simulink model "LoadControl_rev4p2"  (R2024a)
settings: Solver=ode1  StartTime=0.0  StopTime=300  FixedStep=0.001  RelTol=1e-3
undefined symbols (not defined in the file): guxai, K, omega
libraries: SignalEditorBlockLib x2
settings Model: Creator=Hajime.Kondo  LastModifiedBy=Hajime.Kondo

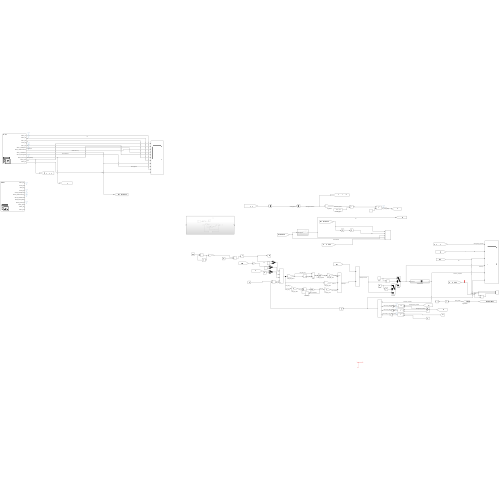
[thumbnail: Simulink's stored preview of the top-level diagram]
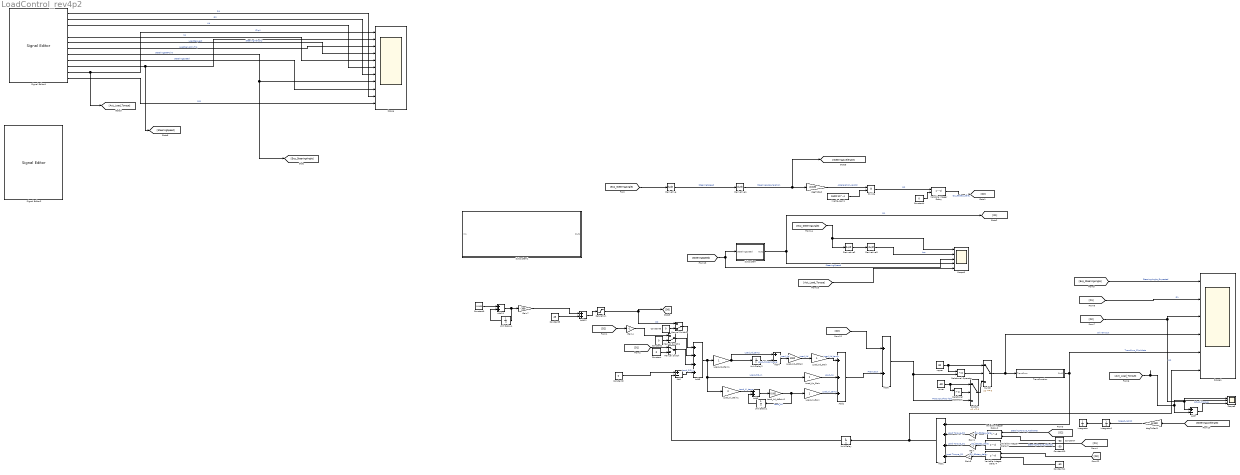
== system LoadControl_rev4p2 ==
  Add : Sum  Inputs=+-
  Add1 : Sum  Inputs=++++
  Add{3,6,11..12} (4 alike) : Sum
  Add2 : Sum  Inputs=+++
  Add4 : Sum  Inputs=+-
  Add5 : Sum  Inputs=++++
  Add7 : Sum  Inputs=+-
  Constant{,1..2,4,6} (5 alike) : Constant  Value=0
  Constant10 : Constant  Value=-50
  Constant11 : Constant  Value=-50
  Constant7 : Constant  Value=-50
  Constant8 : Constant  Value=46
  Constant9 : Constant  Value=0.001
  Derivative{,1..3} (4 alike) : Derivative
  Divide : Product  Inputs=**
  Gain{,1,4..5} (4 alike) : Gain  Gain=-1
  Gain7 : Gain  Gain=-368
  Inertia_kgm1 : Constant  Value=1500*10^-4
  Integrator : Integrator
  Integrator1 : Integrator
  Load_Kd_Gain : Gain
  Load_Kd_Gain1 : Gain
  Load_Kd_dtGain : Gain  Gain=1000
  Load_Kd_dtGain2 : Gain  Gain=0.001
  Load_Ki_Gain : Gain
  Load_Ki_Gain1 : Gain  Gain=0
  Load_Kp_Gain : Gain
  Lower : Constant  Value=-80
  Manual Switch : ManualSwitch
  Manual Switch1 : ManualSwitch  CurrentSetting=0
  Manual Switch2 : ManualSwitch  CurrentSetting=0
  Relational Operator : RelationalOperator  Operator=<=  OutDataTypeStr=boolean  RndMeth=Simplest  InputSameDT=off
  Relational Operator1 : RelationalOperator  OutDataTypeStr=boolean  RndMeth=Simplest  InputSameDT=off
  Saturation : Saturate  UpperLimit=inf  LowerLimit=0
  Scope : Scope  NumInputPorts=11
  Scope1 : Scope  NumInputPorts=6
  Scope3 : Scope  NumInputPorts=5
  Scope6 : Scope  NumInputPorts=3
  Signal Editor1 : SignalEditorBlockLib/Signal Editor  FileName=Simfile.mat  ActiveScenario=SC_rev2  ActiveSignal=data17_D1  IsBus=off  OutputBusObjectStr=Bus: BusObject  SampleTime=0  Interpolate=off  ZeroCross=off  OutputAfterFinalValue=Setting to zero  Unit=inherit  PreserveSignalName=on  ApplySigPropsToAllScenarios=on  ApplySigPropsToAllSignals=off
  Signal Editor2 : SignalEditorBlockLib/Signal Editor  FileName=Simfile.mat  ActiveScenario=SC_rev1  ActiveSignal=data16_Kd  IsBus=off  OutputBusObjectStr=Bus: BusObject  SampleTime=0  Interpolate=off  ZeroCross=off  OutputAfterFinalValue=Setting to zero  Unit=inherit  PreserveSignalName=on  ApplySigPropsToAllScenarios=on  ApplySigPropsToAllSignals=off
  Subsystem : Subsystem
  Subsystem1 : Subsystem
  Switch : Switch  Criteria=u2 ~= 0  SaturateOnIntegerOverflow=off  InputSameDT=off
  Switch1 : Switch  Criteria=u2 ~= 0  SaturateOnIntegerOverflow=off  InputSameDT=off
  TransFunction : Subsystem
  Unit Delay{,1..2,4} (4 alike) : UnitDelay  SampleTime=-1  HasFrameUpgradeWarning=on
  Variable Integer Delay{,2..4} (4 alike) : Delay  DelayLengthSource=Input port
      settings: InputPortMap=u0,p1
  degToRad : Gain  Gain=pi/180
  degToRad1 : Gain  Gain=pi/180
  upper : Constant  Value=80
  wires:
  Signal Editor1/2 -> Scope/7  "D2"
  Signal Editor1/5 -> Scope/5  "Kp"
  Signal Editor1/6 -> Scope/4  "LoadRequest"
  Signal Editor1/7 -> Scope/3  "LoadServoDrvTrq"
  Signal Editor1/10 -> Scope/2, [SteeringSpeed]  "SteeringVelocity"
  Signal Editor1/11 -> [Act_Load_Torque], Scope/1  "ClipX"
  Signal Editor1/8 -> [Exp_SteeringAngle], Scope/8  "SteeringSetPoint"
  Signal Editor1/9 -> Scope/9  "SteeringSpeed"
  ? -> ?
  Variable Integer Delay/1 -> [D2]  "D2_80step_delay"
  [Exp_SteeringAngle] -> Derivative/1
  Add4/1 -> Load_Kd_dtGain/1  "Load_Kd"
  Load_Kp_Gain/1 -> Add2/2  "Load_Kp"
  Lower/1 -> Switch1/1, Relational Operator1/1
  Add3/1 -> Load_Kd_dtGain2/1
  Constant2/1 -> Add/1
  Subsystem/1(Out1) -> Scope3/4, [D1]  "D1"
  Load_Kd_dtGain/1 -> Load_Kd_Gain/1  "Load_Kd"
  Unit Delay/1 -> Add/2
  Relational Operator/1 -> Switch/2
  Manual Switch/1 -> Add5/3
  TransFunction/1(Out1) -> Scope1/5, Add1/1  "TransFunc_ClipXdata"
  Switch1/1 -> Switch/3
  Switch/1 -> Scope1/4, TransFunction/1(TransFunc)  "DriverInput"
  [D2] -> Variable Integer Delay2/1  "SteeringTorque_Acelerate"
  upper/1 -> Switch/1, Relational Operator/1
  Unit Delay2/1 -> Add4/2  "Load_Kd_temp_pre"
  [D2] -> Gain4/1
  [D1] -> Manual Switch/1
  Constant1/1 -> Manual Switch1/2
  [D1] -> Scope1/2  "D1"
  Gain1/1 -> Add1/2  "Load Torque_D2"
  Load_Kd_dtGain2/1 -> Load_Ki_Gain/1, Unit Delay1/1  "Load_Kd"
  Inertia_kgm1/1 -> Divide/2
  Gain/1 -> Add1/3  "Load Torque_D1"
  Add5/1 -> Load_Ki_Gain1/1, Load_Kp_Gain/1, Load_Kd_Gain1/1  "Load_PID_In"
  Integrator1/1 -> Integrator/1
  Unit Delay1/1 -> Add3/2
  [SteeringAcelerate] -> degToRad1/1
  Add7/1 -> Scope6/3
  [Exp_SteeringAngle] -> Scope1/1  "SteeringAngle_Expected"
  Constant8/1 -> Add12/2
  Gain4/1 -> Manual Switch1/1
  Derivative1/1 -> [SteeringAcelerate], degToRad/1  "SteeringAccewleration"
  [D1] -> Variable Integer Delay3/1  "SteeringTorque_Velocity"
  Constant9/1 -> Add11/1
  Gain7/1 -> Add12/1
  degToRad/1 -> Divide/1  "Acceleration_rad/s2"
  Load_Kd_Gain1/1 -> Add4/1, Unit Delay2/1  "Load_Kd_temp"
  Add12/1 -> Saturation/1
  Variable Integer Delay3/1 -> Gain/1  "D2_80step_delay"
  Unit Delay4/1 -> Add11/2
  Load_Ki_Gain/1 -> Add2/3  "Load_Ki_temp"
  degToRad1/1 -> Integrator1/1  "Speed_rad/s2"
  Load_Kd_Gain/1 -> Add2/1  "Load_Kd_temp"
  Constant10/1 -> Variable Integer Delay3/2
  Divide/1 -> Variable Integer Delay/1  "D2"
  Constant7/1 -> Variable Integer Delay2/2
  Variable Integer Delay2/1 -> Gain1/1  "D2_80step_delay"
  Variable Integer Delay4/1 -> Gain5/1  "D2_80step_delay"
  Gain5/1 -> Add1/4  "Load Torque_D1"
  [D0] -> Variable Integer Delay4/1
  Manual Switch1/1 -> Add5/2
  Constant6/1 -> Manual Switch2/2
  Constant11/1 -> Variable Integer Delay4/2
  Add/1 -> Add5/4  "Load_PID_In"
  [Act_Load_Torque] -> Add7/2, Scope6/2  "Actual_Torque"
  Manual Switch2/1 -> Add5/1
  Load_Ki_Gain1/1 -> Add3/1  "Load_Ki_temp"
  Add1/1 -> Scope1/6, Unit Delay/1
  Add11/1 -> Unit Delay4/1, Gain7/1
  Constant/1 -> Manual Switch/2
  [D2] -> Add7/1, Scope6/1, Scope1/3  "D2"
  Relational Operator1/1 -> Switch1/2
  Constant4/1 -> Variable Integer Delay/2
  Saturation/1 -> Manual Switch2/1, [D0]  "D0"
  Add2/1 -> Add6/2  "PIDoutput"
  Add6/1 -> Switch1/3, Relational Operator/2  "PIDoutput+D1+D2"
  [D2] -> Add6/1
  Derivative/1 -> Derivative1/1  "SteeringSpeed"
  [SteeringSpeed] -> Scope3/3, Subsystem/1(SteeringSpeed)  "SteeringSpeed"
  [Act_Load_Torque] -> Scope3/5
  Derivative2/1 -> Derivative3/1
  [Exp_SteeringAngle] -> Derivative2/1, Scope3/1
  Derivative3/1 -> Scope3/2  "Acc"
  Signal Editor1/1 -> Scope/10  "D1"
  Signal Editor1/12 -> Scope/11  "PID"
  Signal Editor1/3 -> Scope/6  "Kd"

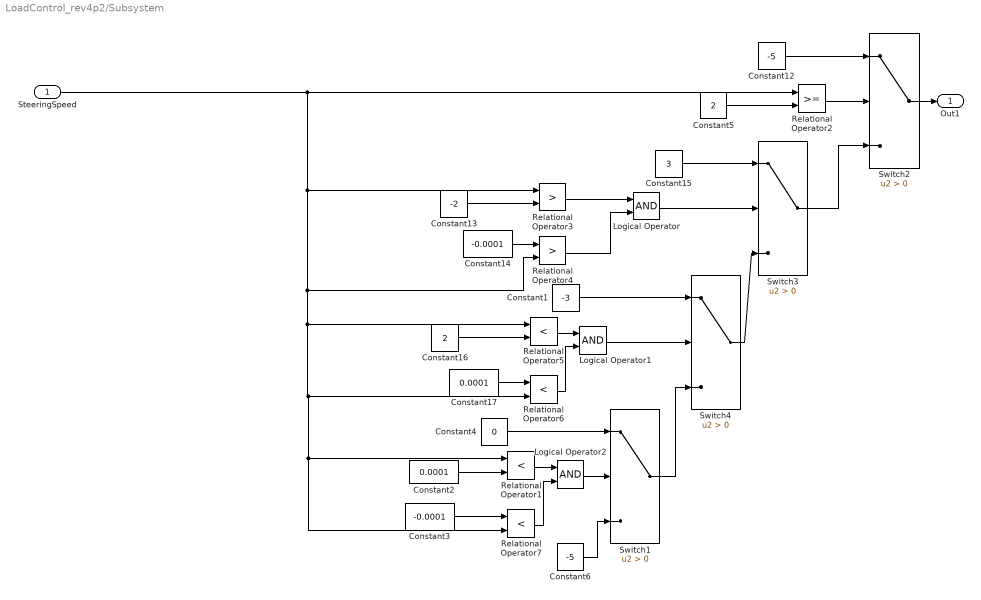
== system LoadControl_rev4p2/Subsystem ==
  SteeringSpeed : Inport
  Constant1 : Constant  Value=-3
  Constant12 : Constant  Value=-5
  Constant13 : Constant  Value=-2
  Constant14 : Constant  Value=-0.0001
  Constant15 : Constant  Value=3
  Constant16 : Constant  Value=2
  Constant17 : Constant  Value=0.0001
  Constant2 : Constant  Value=0.0001
  Constant3 : Constant  Value=-0.0001
  Constant4 : Constant  Value=0
  Constant5 : Constant  Value=2
  Constant6 : Constant  Value=-5
  Logical Operator : Logic  AllPortsSameDT=off  OutDataTypeStr=boolean
  Logical Operator1 : Logic  AllPortsSameDT=off  OutDataTypeStr=boolean
  Logical Operator2 : Logic  AllPortsSameDT=off  OutDataTypeStr=boolean
  Relational Operator{1,5..7} (4 alike) : RelationalOperator  Operator=<  OutDataTypeStr=boolean  RndMeth=Simplest  InputSameDT=off
  Relational Operator2 : RelationalOperator  OutDataTypeStr=boolean  RndMeth=Simplest  InputSameDT=off
  Relational Operator3 : RelationalOperator  Operator=>  OutDataTypeStr=boolean  RndMeth=Simplest  InputSameDT=off
  Relational Operator4 : RelationalOperator  Operator=>  OutDataTypeStr=boolean  RndMeth=Simplest  InputSameDT=off
  Switch{1..4} (4 alike) : Switch  Criteria=u2 > Threshold  SaturateOnIntegerOverflow=off  InputSameDT=off
  Out1 : Outport
  wires:
  Relational Operator4/1 -> Logical Operator/2
  Relational Operator2/1 -> Switch2/2
  Constant17/1 -> Relational Operator6/1
  Logical Operator/1 -> Switch3/2
  Constant12/1 -> Switch2/1
  Constant14/1 -> Relational Operator4/1
  Switch3/1 -> Switch2/3
  Constant15/1 -> Switch3/1
  Relational Operator6/1 -> Logical Operator1/2
  Constant16/1 -> Relational Operator5/2
  Logical Operator1/1 -> Switch4/2
  Relational Operator5/1 -> Logical Operator1/1
  Constant5/1 -> Relational Operator2/2
  Switch4/1 -> Switch3/3
  Relational Operator3/1 -> Logical Operator/1
  Constant13/1 -> Relational Operator3/2
  Constant1/1 -> Switch4/1
  Switch2/1 -> Out1/1
  Relational Operator1/1 -> Logical Operator2/1
  Constant2/1 -> Relational Operator1/2
  Relational Operator7/1 -> Logical Operator2/2
  Constant3/1 -> Relational Operator7/1
  SteeringSpeed/1 -> Relational Operator2/1, Relational Operator3/1, Relational Operator4/2, Relational Operator6/2, Relational Operator7/2, Relational Operator1/1, Relational Operator5/1
  Switch1/1 -> Switch4/3
  Constant4/1 -> Switch1/1
  Logical Operator2/1 -> Switch1/2
  Constant6/1 -> Switch1/3

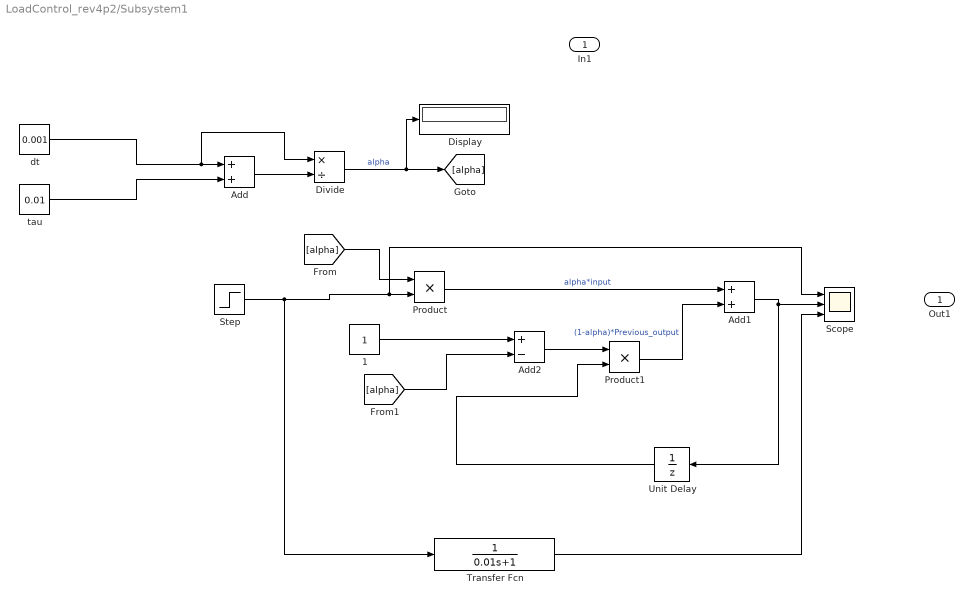
== system LoadControl_rev4p2/Subsystem1 ==
  In1 : Inport
  1 : Constant
  Add : Sum
  Add1 : Sum
  Add2 : Sum  Inputs=+-
  Display : Display
  Divide : Product  Inputs=*/
  Product : Product
  Product1 : Product
  Scope : Scope  NumInputPorts=3
  Step : Step  SampleTime=0
  Transfer Fcn : TransferFcn  Denominator=[0.01 1]
  Unit Delay : UnitDelay  SampleTime=-1  HasFrameUpgradeWarning=on
  dt : Constant  Value=0.001
  tau : Constant  Value=0.01
  Out1 : Outport
  wires:
  dt/1 -> Divide/1, Add/1
  tau/1 -> Add/2
  Add/1 -> Divide/2
  Step/1 -> Transfer Fcn/1, Scope/1, Product/2
  Divide/1 -> Display/1, [alpha]  "alpha"
  Product/1 -> Add1/1  "alpha*input"
  Unit Delay/1 -> Product1/2
  Add2/1 -> Product1/1
  1/1 -> Add2/1
  [alpha] -> Product/1
  [alpha] -> Add2/2
  Product1/1 -> Add1/2  "(1-alpha)*Previous_output"
  Add1/1 -> Unit Delay/1, Scope/2
  Transfer Fcn/1 -> Scope/3

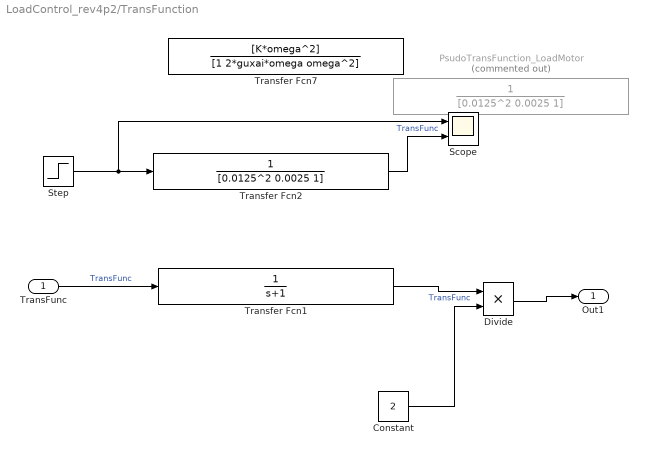
== system LoadControl_rev4p2/TransFunction ==
  TransFunc : Inport
  Constant : Constant  Value=2
  Divide : Product  Inputs=**
  PsudoTransFunction_LoadMotor : TransferFcn  Commented=on  Denominator=[0.0125^2 0.0025 1]
  Scope : Scope  NumInputPorts=2
  Step : Step  After=50  SampleTime=0
  Transfer Fcn1 : TransferFcn  Denominator=[1 1]
  Transfer Fcn2 : TransferFcn  Denominator=[0.0125^2 0.0025 1]
  Transfer Fcn7 : TransferFcn  Numerator=[K*omega^2]  Denominator=[1 2*guxai*omega omega^2]
  Out1 : Outport
  wires:
  TransFunc/1 -> Transfer Fcn1/1  "TransFunc"
  Constant/1 -> Divide/2
  Transfer Fcn1/1 -> Divide/1  "TransFunc"
  Divide/1 -> Out1/1
  Step/1 -> Scope/1, Transfer Fcn2/1
  Transfer Fcn2/1 -> Scope/2  "TransFunc"
